simulink model "CTDSM_CRFF_SECOND_2048_WITH_ELD_COMPENSATION"  (R2025b)
settings: Solver=VariableStepAuto  StartTime=0.0  StopTime=0.5  RelTol=1e-3
undefined symbols (not defined in the file): Kc
libraries: simulink_extras x1
settings Model: Creator=Team_33  LastModifiedBy=k2vas

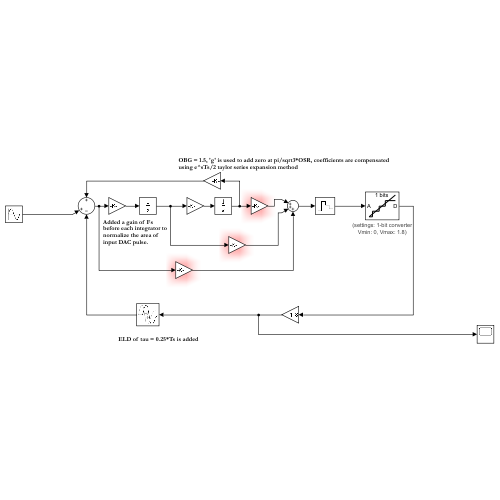
[thumbnail: Simulink's stored preview of the top-level diagram]
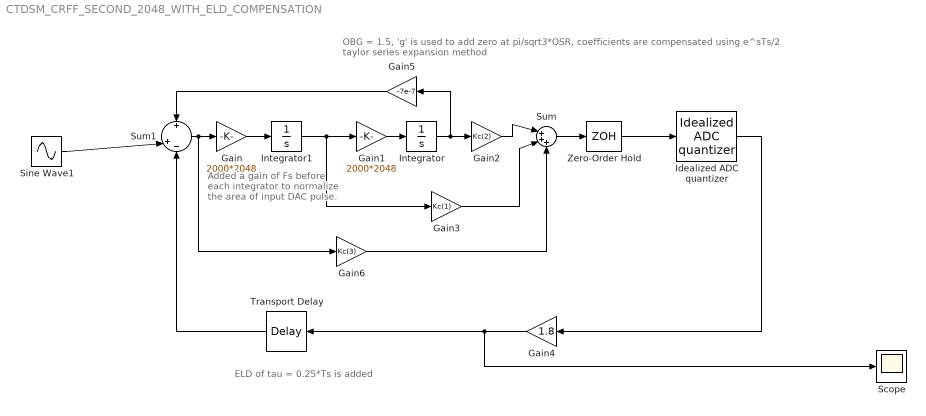
== system CTDSM_CRFF_SECOND_2048_WITH_ELD_COMPENSATION ==
  note: OBG = 1.5, 'g' is used to add zero at pi/sqrt3*OSR, coefficients are compensated using e^sTs/2 taylor series expansion method
  note: ELD of tau = 0.25*Ts is added
  note: Added a gain of Fs before each integrator to normalize the area of input DAC pulse.
  Gain : Gain  Gain=2000*2048
  Gain1 : Gain  Gain=2000*2048
  Gain2 : Gain  Gain=Kc(2)
  Gain3 : Gain  Gain=Kc(1)
  Gain4 : Gain  Gain=1.8
  Gain5 : Gain  Gain=-7e-7
  Gain6 : Gain  Gain=Kc(3)
  Idealized ADC quantizer : simulink_extras/Additional Discrete/Idealized ADC quantizer  NumberOfConverterBits=1  Vmin=0  Vmax=1.8  OutputDataType=double  OutputNegativeValues=off
  Integrator : Integrator
  Integrator1 : Integrator
  Scope : Scope
      settings: ActiveDisplayYMinimum=-0.225  ActiveDisplayYMaximum=2.025  DataLoggingVariableName=output_data  DataLoggingSaveFormat=Array
  Sine Wave1 : Sin  Amplitude=0.5  Bias=0.9  Frequency=((2000*1024)*127*2*2*pi)/(32768*32)  SampleTime=0
  Sum : Sum  Inputs=|+++
  Sum1 : Sum  Inputs=+|+-
  Transport Delay : TransportDelay  DelayTime=1/(2000*2048*4)
  Zero-Order Hold : ZeroOrderHold  SampleTime=1/(2000*1024*2)
  wires:
  Zero-Order Hold/1 -> Idealized ADC quantizer/1
  Integrator/1 -> Gain5/1, Gain2/1
  Sum/1 -> Zero-Order Hold/1
  Gain2/1 -> Sum/1
  Gain3/1 -> Sum/2
  Sum1/1 -> Gain6/1, Gain/1
  Integrator1/1 -> Gain3/1, Gain1/1
  Gain/1 -> Integrator1/1
  Gain1/1 -> Integrator/1
  Sine Wave1/1 -> Sum1/2
  Gain5/1 -> Sum1/1
  Gain6/1 -> Sum/3
  Idealized ADC quantizer/1 -> Gain4/1
  Gain4/1 -> Transport Delay/1, Scope/1
  Transport Delay/1 -> Sum1/3
